simulink model "motor_model"  (R2020b)
settings: Solver=VariableStepAuto  StartTime=0.0  StopTime=10.0  RelTol=1e-3
values from neighbouring files (symbols this model uses):
  a = 12.5    [Rocky_closed_loop_poles.m]    (also in load_values.m; rocky_calibration.m = 1/(right_time_constant))
  b = 0.00323    [Rocky_closed_loop_poles.m]    (also in load_values.m; rocky_calibration.m = right_K)
  Ci = double(solutions.Ci)    [Rocky_closed_loop_poles.m]    (also in load_values.m = 659)
  JiCp = 598    [load_values.m]
  Jp = double(solutions.Jp)    [Rocky_closed_loop_poles.m]    (also in load_values.m = -12.38)
settings Model: Creator=wsh32  LastModifiedBy=wsh32

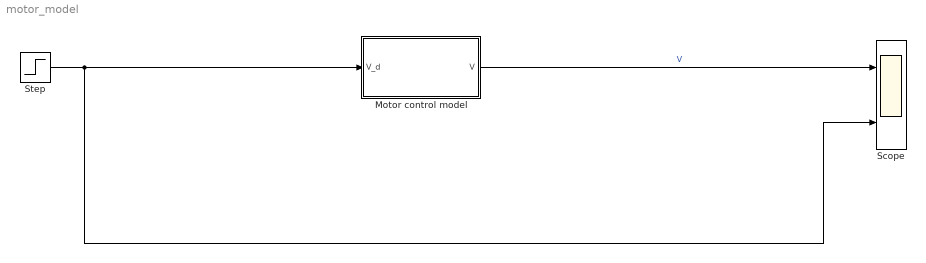
== system motor_model ==
  Motor control model : Subsystem
  Scope : Scope  NumInputPorts=2
  Step : Step  SampleTime=0
  wires:
  Step/1 -> Motor control model/1(V_d), Scope/2
  Motor control model/1(V) -> Scope/1  "V"

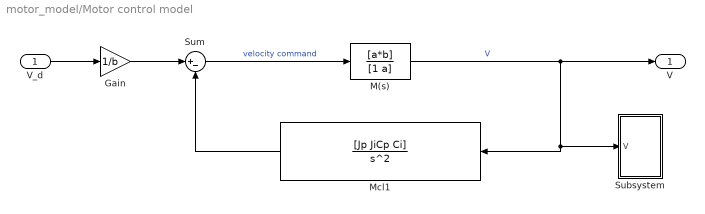
== system motor_model/Motor control model ==
  V_d : Inport
  Gain : Gain  Gain=1/b
  M(s) : TransferFcn  Numerator=[a*b]  Denominator=[1 a]
  Mcl1 : TransferFcn  Numerator=[Jp JiCp Ci]  Denominator=[1 0 0]
  Subsystem : Subsystem
  Sum : Sum  Inputs=|+-
  V : Outport
  wires:
  Sum/1 -> M(s)/1  "velocity command"
  V_d/1 -> Gain/1
  M(s)/1 -> V/1, Mcl1/1, Subsystem/1(V)  "V"
  Mcl1/1 -> Sum/2
  Gain/1 -> Sum/1

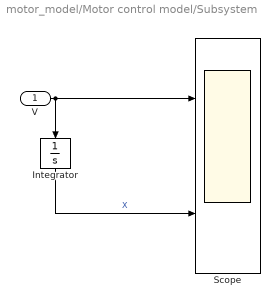
== system motor_model/Motor control model/Subsystem ==
  V : Inport
  Integrator : Integrator
  Scope : Scope  NumInputPorts=2
  wires:
  V/1 -> Integrator/1, Scope/1
  Integrator/1 -> Scope/2  "X"
